simulink model "half_car_passive_model"  (R2018a)
settings: Solver=ode23t  StartTime=0.0  StopTime=5  MaxStep=0.001  RelTol=1e-3
values from neighbouring files (symbols this model uses):
  a = 0.675    [parameters.m]
  b = 0.6    [parameters.m]
  b1 = 3000    [parameters.m]
  b2 = 3000    [parameters.m]
  J = 48.96    [parameters.m]
  k1 = 190000    [parameters.m]
  k2 = 190000    [parameters.m]
  k3 = 16000    [parameters.m]
  k4 = 24000    [parameters.m]
  ms = 105    [parameters.m]
  mu_f = 25    [parameters.m]
  mu_r = 30    [parameters.m]
  td = L/(v*5/18)    (= 0.2655)    [parameters.m]
libraries: sdolib x2, simulink x2
settings Model: Creator=Saurabh Suman  LastModifiedBy=Saurabh Suman

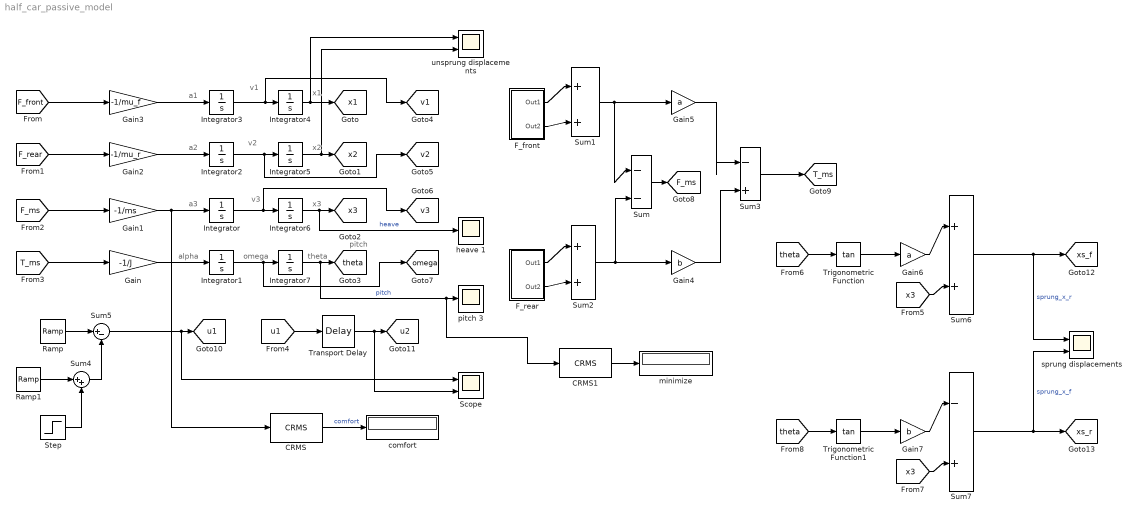
== system half_car_passive_model ==
  note: pitch
  note: x1
  note: x2
  note: x3
  note: theta
  note: a1
  note: a2
  note: a3
  note: alpha
  note: omega
  note: v3
  note: v2
  note: v1
  CRMS : sdolib/RMS Blocks/CRMS
      settings: SourceProductName=Simulink Design Optimization  SourceProductBaseCode=SO
  CRMS1 : sdolib/RMS Blocks/CRMS
      settings: SourceProductName=Simulink Design Optimization  SourceProductBaseCode=SO
  F_front : Subsystem
  F_rear : Subsystem
  Gain : Gain  Gain=-1/J
  Gain1 : Gain  Gain=-1/ms
  Gain2 : Gain  Gain=-1/mu_r
  Gain3 : Gain  Gain=-1/mu_f
  Gain4 : Gain  Gain=b
  Gain5 : Gain  Gain=a
  Gain6 : Gain  Gain=a
  Gain7 : Gain  Gain=b
  Integrator{,1..7} (8 alike) : Integrator
  Ramp : simulink/Sources/Ramp  slope=0.5  start=1  InitialOutput=0
  Ramp1 : simulink/Sources/Ramp  slope=0.5  start=1.3  InitialOutput=0
  Scope : Scope  NumInputPorts=2
  Step : Step  Time=1.3  After=0.15  SampleTime=0
  Sum : Sum  Inputs=|--
  Sum{1..2,4,6} (4 alike) : Sum  Inputs=|++
  Sum3 : Sum  Inputs=|-+
  Sum5 : Sum  Inputs=|+-
  Sum7 : Sum  Inputs=|-+
  Transport Delay : TransportDelay  DelayTime=td
  Trigonometric Function : Trigonometry  Operator=tan  OutputSignalType=real
  Trigonometric Function1 : Trigonometry  Operator=tan  OutputSignalType=real
  comfort : Display
  heave 1 : Scope
  minimize : Display
  pitch 3 : Scope
  sprung displacements : Scope  NumInputPorts=2
  unsprung displacements : Scope  NumInputPorts=2
  tag scope: F_ms=global, T_ms=global, omega=global, theta=global, u1=global, u2=global, v1=global, v2=global, v3=global, x1=global, x2=global, x3=global, xs_f=global, xs_r=global
  wires:
  Integrator3/1 -> [v1], Integrator4/1
  Integrator2/1 -> [v2], Integrator5/1
  Integrator/1 -> [v3], Integrator6/1
  Integrator1/1 -> [omega], Integrator7/1
  Gain/1 -> Integrator1/1
  Gain3/1 -> Integrator3/1
  Gain2/1 -> Integrator2/1
  Integrator6/1 -> heave 1/1, [x3]  "heave"
  Integrator7/1 -> CRMS1/1, pitch 3/1, [theta]  "pitch"
  [F_front] -> Gain3/1
  [F_rear] -> Gain2/1
  [F_ms] -> Gain1/1
  [T_ms] -> Gain/1
  F_front/1(Out1) -> Sum1/1
  F_front/2(Out2) -> Sum1/2
  F_rear/1(Out1) -> Sum2/1
  F_rear/2(Out2) -> Sum2/2
  Sum/1 -> [F_ms]
  Sum1/1 -> Sum/1, Gain5/1
  Sum2/1 -> Sum/2, Gain4/1
  Sum3/1 -> [T_ms]
  Gain5/1 -> Sum3/1
  Gain4/1 -> Sum3/2
  Step/1 -> Sum4/2
  Transport Delay/1 -> Scope/2, [u2]
  [u1] -> Transport Delay/1
  CRMS/1 -> comfort/1  "comfort"
  Ramp1/1 -> Sum4/1
  Sum4/1 -> Sum5/2
  Gain1/1 -> CRMS/1, Integrator/1
  Sum5/1 -> Scope/1, [u1]
  Ramp/1 -> Sum5/1
  Integrator5/1 -> unsprung displacements/2, [x2]
  Integrator4/1 -> unsprung displacements/1, [x1]
  Trigonometric Function/1 -> Gain6/1
  [theta] -> Trigonometric Function/1
  [x3] -> Sum6/2
  Gain6/1 -> Sum6/1
  Sum6/1 -> sprung displacements/1, [xs_f]  "sprung_x_r"
  Trigonometric Function1/1 -> Gain7/1
  Gain7/1 -> Sum7/1
  Sum7/1 -> sprung displacements/2, [xs_r]  "sprung_x_f"
  [theta] -> Trigonometric Function1/1
  [x3] -> Sum7/2
  CRMS1/1 -> minimize/1

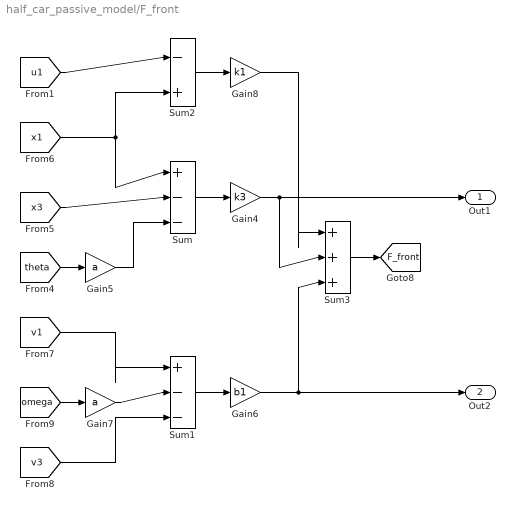
== system half_car_passive_model/F_front ==
  Gain4 : Gain  Gain=k3
  Gain5 : Gain  Gain=a
  Gain6 : Gain  Gain=b1
  Gain7 : Gain  Gain=a
  Gain8 : Gain  Gain=k1
  Sum : Sum  Inputs=|+--
  Sum1 : Sum  Inputs=|+--
  Sum2 : Sum  Inputs=|-+
  Sum3 : Sum  Inputs=|+++
  Out1 : Outport
  Out2 : Outport  Port=2
  tag scope: F_front=global
  wires:
  [v3] -> Sum1/3
  [theta] -> Gain5/1
  Sum/1 -> Gain4/1
  [u1] -> Sum2/1
  Sum1/1 -> Gain6/1
  Gain5/1 -> Sum/3
  Gain4/1 -> Out1/1, Sum3/2
  Gain8/1 -> Sum3/1
  Gain6/1 -> Out2/1, Sum3/3
  Sum2/1 -> Gain8/1
  [v1] -> Sum1/1
  [x1] -> Sum/1, Sum2/2
  [x3] -> Sum/2
  Sum3/1 -> [F_front]
  [omega] -> Gain7/1
  Gain7/1 -> Sum1/2

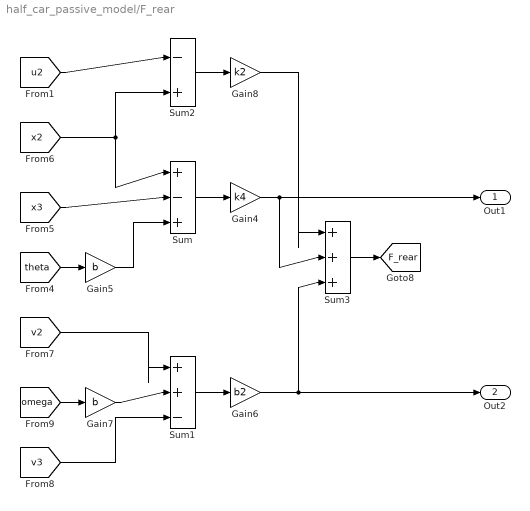
== system half_car_passive_model/F_rear ==
  Gain4 : Gain  Gain=k4
  Gain5 : Gain  Gain=b
  Gain6 : Gain  Gain=b2
  Gain7 : Gain  Gain=b
  Gain8 : Gain  Gain=k2
  Sum : Sum  Inputs=|+-+
  Sum1 : Sum  Inputs=|++-
  Sum2 : Sum  Inputs=|-+
  Sum3 : Sum  Inputs=|+++
  Out1 : Outport
  Out2 : Outport  Port=2
  tag scope: F_rear=global
  wires:
  Gain6/1 -> Out2/1, Sum3/3
  Sum2/1 -> Gain8/1
  Sum3/1 -> [F_rear]
  [x3] -> Sum/2
  Gain4/1 -> Out1/1, Sum3/2
  [omega] -> Gain7/1
  [x2] -> Sum/1, Sum2/2
  [v2] -> Sum1/1
  [u2] -> Sum2/1
  [theta] -> Gain5/1
  Gain5/1 -> Sum/3
  Gain8/1 -> Sum3/1
  Sum/1 -> Gain4/1
  [v3] -> Sum1/3
  Sum1/1 -> Gain6/1
  Gain7/1 -> Sum1/2
